simulink model "Control_Induction_Motor_by_3phaseinverter_120D_Conduction"  (R2021b)
settings: Solver=VariableStepAuto  StartTime=0.0  StopTime=2  RelTol=1e-3
libraries: spsMosfetLib x6, spsVoltageMeasurementLib x3, spsDCVoltageSourceLib x1, spsAsynchronousMachineSIUnitsLib x1, spspowerguiLib x1
settings Model: Creator=Vansh  LastModifiedBy=Vansh

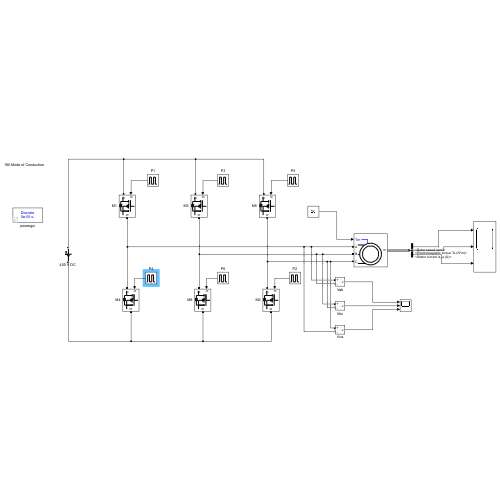
[thumbnail: Simulink's stored preview of the top-level diagram]
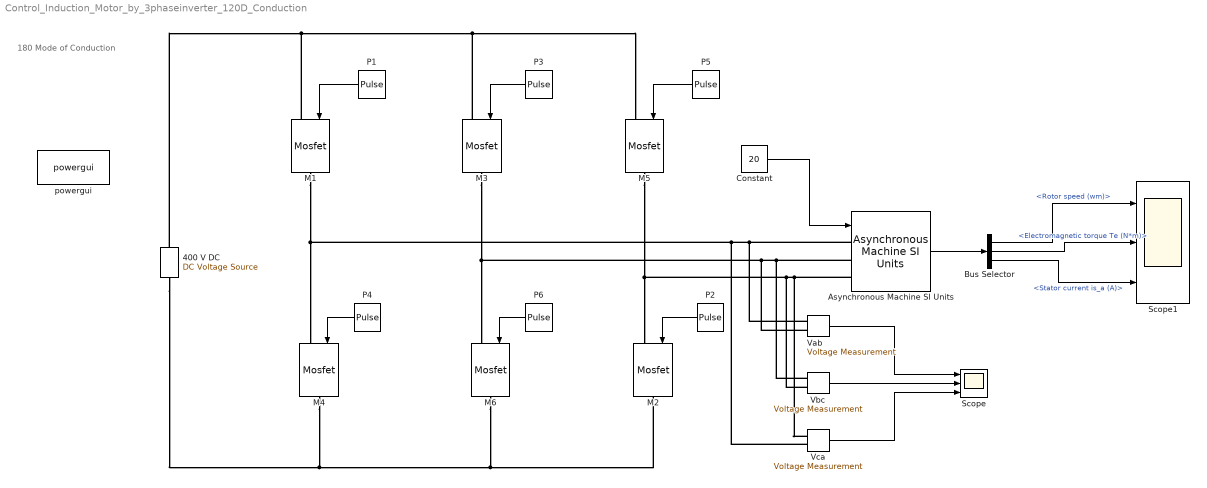
== system Control_Induction_Motor_by_3phaseinverter_120D_Conduction ==
  note: 180 Mode of Conduction
  "400 V DC " : spsDCVoltageSourceLib/DC Voltage Source  Amplitude=400  Measurements=None
  Asynchronous Machine SI Units : spsAsynchronousMachineSIUnitsLib/Asynchronous Machine SI Units  RotorType=Squirrel-cage  PresetModel="15:  5.4 HP (4KW)   400 V  50Hz 1430 RPM"  MechanicalLoad=Torque Tm  ShowDetailedParameters=on  ReferenceFrame=Rotor  Units=SI  MeasurementBus=off  NominalParameters=[4000 400 50]  VoltageRatio=1  Stator=[1.405 0.005839]  Rotor=[1.395 0.005839]  Cage1=[0.4155 0.002066]  Cage2=[0.4168 0.0003495]  Lm=0.1722  Mechanical=[0.0131 0.002985 2]  PolePairs=2  InitialConditions=[0 0 0 0 0 0 0 0]  SimulateSaturation=off  Saturation=[14.03593122, 27.81365428, 53.79336849, 72.68890987, 97.98006896, 148.6815601, 215.7428561, 302.9841135, 428.7778367 ; 230, 322, 414, 460, 506, 552, 598, 644, 690]  LoadFlowParameters=1492000  TsPowergui=0  TsBlock=-1  IterativeModel=Trapezoidal non iterative  IterativeDiscreteModel=Trapezoidal non iterative  Pmec=1.492e+006
  Bus Selector : BusSelector  OutputSignals=Mechanical.Rotor speed (wm),Mechanical.Electromagnetic torque Te (N*m),Stator measurements.Stator current is_a (A)
  Constant : Constant  Value=20
  M{1..6} (6 alike) : spsMosfetLib/Mosfet  Ron=0.1  Lon=0  Rd=0.01  Vfd=0  IC=0  Rs=1e5  Cs=inf  Measurements=off
  P1 : DiscretePulseGenerator  PulseType=Time based  Period=1/50  PulseWidth=33.333
  P2 : DiscretePulseGenerator  PulseType=Time based  Period=1/50  PulseWidth=33.333  PhaseDelay=60*(20e-3/360)
  P3 : DiscretePulseGenerator  PulseType=Time based  Period=1/50  PulseWidth=33.333  PhaseDelay=120*(20e-3/360)
  P4 : DiscretePulseGenerator  PulseType=Time based  Period=1/50  PulseWidth=33.333  PhaseDelay=180*(20e-3/360)
  P5 : DiscretePulseGenerator  PulseType=Time based  Period=1/50  PulseWidth=33.333  PhaseDelay=240*(20e-3/360)
  P6 : DiscretePulseGenerator  PulseType=Time based  Period=1/50  PulseWidth=33.333  PhaseDelay=300*(20e-3/360)
  Scope : Scope  NumInputPorts=3
  Scope1 : Scope  NumInputPorts=3
  Vab : spsVoltageMeasurementLib/Voltage Measurement  PhasorSimulation=off  OutputType=Complex  PSBequivalent=0
  Vbc : spsVoltageMeasurementLib/Voltage Measurement  PhasorSimulation=off  OutputType=Complex  PSBequivalent=0
  Vca : spsVoltageMeasurementLib/Voltage Measurement  PhasorSimulation=off  OutputType=Complex  PSBequivalent=0
  powergui : spspowerguiLib/powergui  Priority=1  SimulationMode=Discrete  SampleTime=50e-6  frequency=60  Iterations=50  frequencyindice=50  Pbase=100e6  ErrMax=1e-4  UnitsV=kV  UnitsW=MW  buscounter=0  FunctionMessages=off  echomessages=off  EnableUseOfTLC=off  CurrentSourceSwitches=off  DisableSnubberDevices=off  DisableRonSwitches=off  DisableVfSwitches=off  DisplayEquations=off  AutomaticDiscreteSolvers=off  SolverType=Tustin/Backward Euler (TBE)  Interpol=off  ExternalGateDelay=off  methode=off  Ts=100  x0status=blocks  SPID=on  SwTol=0  HookPort=off  NonlinearTolerance=1e-4  nMaxIteration=100  ContinueOnMaxIteration=off  RestoreLinks=warning  ResistiveCurrentMeasurement=off  Frange=[0:2:500]  Ylog=off  Xlog=on  ShowGrid=off  save=off  variable=ZData  structure=0  ZoomFFT=off  StartTime=0.0  cycles=1  DisplayStyle=1  fundamental=60  FreqAxis=off  MaxFrequency=1000  frequencyindicesteady=1  RmsSteady=1  display=off
  wires:
  Asynchronous Machine SI Units/1 -> Bus Selector/1
  P1/1 -> M1/1
  P2/1 -> M2/1
  P3/1 -> M3/1
  P4/1 -> M4/1
  P5/1 -> M5/1
  P6/1 -> M6/1
  Constant/1 -> Asynchronous Machine SI Units/1
  Vab/1 -> Scope/1
  Vbc/1 -> Scope/2
  Vca/1 -> Scope/3
  Bus Selector/1 -> Scope1/1  "<Rotor speed (wm)>"
  Bus Selector/2 -> Scope1/2  "<Electromagnetic torque Te (N*m)>"
  Bus Selector/3 -> Scope1/3  "<Stator current is_a (A)>"
  connections:
  "400 V DC "/RConn1 -- M1/LConn1 -- M3/LConn1 -- M5/LConn1
  "400 V DC "/LConn1 -- M4/RConn1 -- M6/RConn1 -- M2/RConn1
  M1/RConn1 -- Vca/LConn2 -- Vab/LConn1 -- Asynchronous Machine SI Units/LConn1 -- M4/LConn1
  M3/RConn1 -- Vab/LConn2 -- Vbc/LConn1 -- Asynchronous Machine SI Units/LConn2 -- M6/LConn1
  M5/RConn1 -- Vbc/LConn2 -- Vca/LConn1 -- Asynchronous Machine SI Units/LConn3 -- M2/LConn1
